simulink model "xianbolvvo2021b"  (R2021b)
settings: Solver=ode1  StartTime=0.0  StopTime=10  FixedStep=0.001  RelTol=1e-3
undefined symbols (not defined in the file): alldata3K_input, alldata3K_output, alldata5K_input, alldata5K_output, alldata7K_input, alldata7K_output, DiscIntNeverNeededParam, Hzden, Hznum
libraries: eeGeneralControl x7, cstblocks x1
settings Model: Creator=renjianze  LastModifiedBy=renjianze
settings DebuggingCC: UnconnectedInputMsg=none  UnconnectedOutputMsg=none  UnconnectedLineMsg=none
settings ModelReferenceCC: EnableRefExpFcnMdlSchedulingChecks=off
settings RTWCC: DLArmComputeVersion=20.02.1

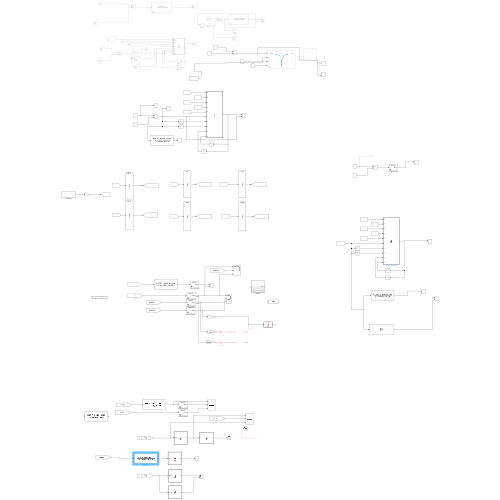
[thumbnail: Simulink's stored preview of the top-level diagram]
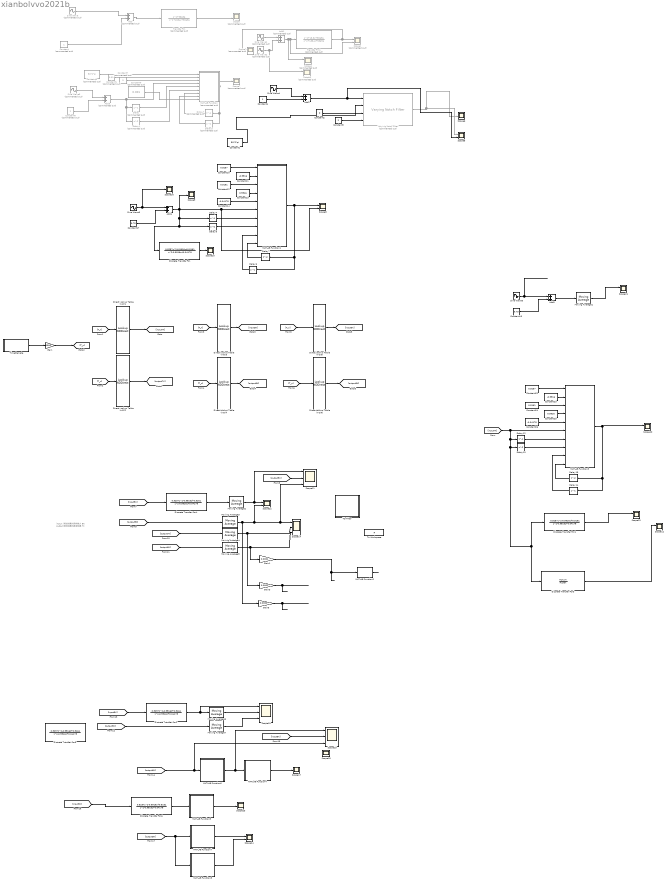
== system xianbolvvo2021b ==
  note: input：测试结果的采样输入 6K
      | output:测试结果的滤波结果  7k
  Add : Sum  Commented=on
  Add1 : Sum  Commented=on
  Add2 : Sum
  Add3 : Sum  Commented=on
  Add4 : Sum
  Add5 : Sum
  Constant : Constant  Commented=on
  Constant1 : Constant  Value=50*2*pi
  Constant10 : Constant  Value=0.5257
  Constant11 : Constant  Value=-0.9916
  Constant12 : Constant  Value=0.5161
  Constant13 : Constant  Value=0.9916
  Constant14 : Constant  Value=-0.04178
  Constant15 : Constant  Value=9.75
  Constant17 : Constant  Value=9.75
  Constant2 : Constant  Value=0
  Constant22 : Constant  Value=0.5257
  Constant23 : Constant  Value=-0.9916
  Constant24 : Constant  Value=0.5161
  Constant25 : Constant  Value=0.9916
  Constant26 : Constant  Value=-0.04178
  Constant3 : Constant  Value=2
  Constant4 : Constant
  Constant5 : Constant  Commented=on  Value=50*2*pi
  Constant6 : Constant  Commented=on  Value=0.01
  Constant7 : Constant  Commented=on  Value=3
  Constant8 : Constant  Commented=on
  Constant9 : Constant  Commented=on  Value=0.001
  Delay : Delay  Commented=on  DelayLength=1
  Delay1 : Delay  Commented=on
  Delay{4,6,12,14} (4 alike) : Delay  DelayLength=1
  Delay{5,7,13,15} (4 alike) : Delay
  Delay2 : Delay  Commented=on  DelayLength=1
  Delay3 : Delay  Commented=on
  Direct Lookup Table (n-D)1 : LookupNDDirect  NumberOfTableDimensions=1  Table=alldata7K_input
  Direct Lookup Table (n-D)2 : LookupNDDirect  NumberOfTableDimensions=1  Table=alldata7K_output
  Direct Lookup Table (n-D)3 : LookupNDDirect  NumberOfTableDimensions=1  Table=alldata5K_input
  Direct Lookup Table (n-D)4 : LookupNDDirect  NumberOfTableDimensions=1  Table=alldata5K_output
  Direct Lookup Table (n-D)5 : LookupNDDirect  NumberOfTableDimensions=1  Table=alldata3K_input
  Direct Lookup Table (n-D)6 : LookupNDDirect  NumberOfTableDimensions=1  Table=alldata3K_output
  Discrete Transfer Fcn{,1..2,4..6} (6 alike) : DiscreteTransferFcn  Numerator=[0.5257 -0.9916 0.5161]  Denominator=[1 -0.9916 0.04178]
  Discrete Transfer Fcn3 : DiscreteTransferFcn  Numerator=Hznum  Denominator=Hzden
  Gain : Gain  Gain=1000
  Gain1 : Gain  Gain=0.0001
  Gain3 : Gain  Gain=0.0001
  Gain5 : Gain  Gain=0.0001
  MATLAB Function : MATLAB Function  Commented=on  TreatAsAtomicUnit=on
  MATLAB Function1 : MATLAB Function  TreatAsAtomicUnit=on
  MATLAB Function2 : MATLAB Function  TreatAsAtomicUnit=on
  MATLAB Function3 : MATLAB Function  TreatAsAtomicUnit=on
  MATLAB Function4 : MATLAB Function  TreatAsAtomicUnit=on
  MATLAB Function5 : MATLAB Function  TreatAsAtomicUnit=on
  MATLAB Function6 : MATLAB Function  TreatAsAtomicUnit=on
  MATLAB Function7 : MATLAB Function  TreatAsAtomicUnit=on
  MATLAB Function8 : MATLAB Function  TreatAsAtomicUnit=on
  Moving Average{1..7} (7 alike) : eeGeneralControl/Moving Average  VariantControl=Variant1  LabelModeActiveChoice=Discrete  f=50  x0=0  BufferSize=8192  Ts=0.001
      settings: SourceProductBaseCode=PS
  Scope{,1..4} (5 alike) : Scope  Commented=on  NumInputPorts=2
  Scope{6,9..10,16..18,23} (7 alike) : Scope
  Scope{11,14..15,19} (4 alike) : Scope  NumInputPorts=3
  Scope{5,8,12..13,20..22,24} (8 alike) : Scope  NumInputPorts=2
  Scope7 : Scope  Commented=on
  Sine Wave : Sin  Commented=on  Amplitude=0.3  Frequency=50*2*pi  SampleTime=0
  Sine Wave1 : Sin  Commented=on  Frequency=50*2*pi  SampleTime=0
  Sine Wave2 : Sin  Commented=on  Frequency=100*2*pi  SampleTime=0
  Sine Wave3 : Sin  Commented=on  Amplitude=0.3  Frequency=50*2*pi  SampleTime=0
  Sine Wave4 : Sin  Amplitude=0.3  Frequency=50*2*pi  SampleTime=0
  Sine Wave5 : Sin  Amplitude=1.25  Frequency=50*2*pi  Phase=pi/2  SampleTime=0
  Sine Wave6 : Sin  Amplitude=1.25  Frequency=50*2*pi  Phase=pi/2  SampleTime=0
  TD Filter : Subsystem
  TimeGenrate : Subsystem
  To Workspace : ToWorkspace  VariableName=R  SampleTime=-1
  Transfer Fcn : TransferFcn  Commented=on  Numerator=[1 0 98696]  Denominator=[1 1884 98696]
  Transfer Fcn1 : TransferFcn  Commented=on  Numerator=[1 18.8 98696]  Denominator=[1 1884 98696]
  Varying Notch Filter : cstblocks/Linear Parameter Varying/Varying Notch Filter  Commented=on
      settings: SourceProductBaseCode=CT
  wires:
  Transfer Fcn/1 -> Scope/2
  Sine Wave/1 -> Add/1
  Constant/1 -> Add/2
  Add/1 -> Transfer Fcn/1
  Sine Wave1/1 -> Add1/1
  Add1/1 -> Scope4/1, Scope1/2, Transfer Fcn1/1
  Transfer Fcn1/1 -> Scope2/1, Scope1/1
  Sine Wave2/1 -> Scope3/1, Add1/2
  Constant1/1 -> Varying Notch Filter/2
  Constant2/1 -> Varying Notch Filter/3
  Constant3/1 -> Varying Notch Filter/4
  Varying Notch Filter/1 -> Scope6/1, Scope5/1
  Sine Wave4/1 -> Add2/1
  Add2/1 -> Scope5/2, Varying Notch Filter/1
  Constant4/1 -> Add2/2
  Constant5/1 -> MATLAB Function/1(freq)
  Constant6/1 -> MATLAB Function/2(gmin)
  Constant7/1 -> MATLAB Function/3(damp)
  Constant8/1 -> Add3/2
  Sine Wave3/1 -> Add3/1
  Add3/1 -> Delay1/1, Delay/1, MATLAB Function/4(x)
  Delay/1 -> MATLAB Function/5(x1)
  Delay1/1 -> MATLAB Function/6(x2)
  MATLAB Function/1(y) -> Delay3/1, Delay2/1, Scope7/1
  Delay2/1 -> MATLAB Function/7(y1)
  Delay3/1 -> MATLAB Function/8(y2)
  Constant9/1 -> MATLAB Function/9(Ts)
  Constant10/1 -> MATLAB Function1/1(a0)
  Constant11/1 -> MATLAB Function1/2(a1)
  Constant12/1 -> MATLAB Function1/3(a2)
  Constant13/1 -> MATLAB Function1/4(b1)
  Constant14/1 -> MATLAB Function1/5(b2)
  Add4/1 -> Scope9/1, Discrete Transfer Fcn/1, Delay5/1, Delay4/1, MATLAB Function1/6(x), Scope8/2
  Sine Wave5/1 -> Scope16/1, Add4/1
  Constant17/1 -> Add4/2
  Delay4/1 -> MATLAB Function1/7(x1)
  Delay5/1 -> MATLAB Function1/8(x2)
  Delay6/1 -> MATLAB Function1/9(y1)
  Delay7/1 -> MATLAB Function1/10(y2)
  MATLAB Function1/1(y) -> Scope8/1, Delay6/1, Delay7/1
  Discrete Transfer Fcn/1 -> Scope10/1
  TimeGenrate/1(t) -> Gain/1
  Gain/1 -> [T_n]
  Direct Lookup Table (n-D)1/1 -> [input7K]
  Direct Lookup Table (n-D)2/1 -> [output7K]
  MATLAB Function3/1(y) -> Scope20/1, Delay15/1, Delay14/1
  Delay15/1 -> MATLAB Function3/10(y2)
  Delay14/1 -> MATLAB Function3/9(y1)
  Delay13/1 -> MATLAB Function3/8(x2)
  Delay12/1 -> MATLAB Function3/7(x1)
  [input7K] -> Delay12/1, Discrete Transfer Fcn1/1, Discrete Transfer Fcn3/1, Delay13/1, MATLAB Function3/6(x)
  Constant26/1 -> MATLAB Function3/5(b2)
  Constant25/1 -> MATLAB Function3/4(b1)
  Constant24/1 -> MATLAB Function3/3(a2)
  Constant23/1 -> MATLAB Function3/2(a1)
  Constant22/1 -> MATLAB Function3/1(a0)
  Discrete Transfer Fcn3/1 -> Scope12/1
  Discrete Transfer Fcn1/1 -> Scope13/1
  Constant15/1 -> Add5/2
  Sine Wave6/1 -> Add5/1
  Add5/1 -> Moving Average1/1
  Moving Average1/1 -> Scope21/1
  Discrete Transfer Fcn4/1 -> Moving Average2/1
  [input5K] -> Discrete Transfer Fcn4/1
  [output5K] -> Moving Average3/1
  Moving Average2/1 -> Scope11/1, Scope22/1
  Moving Average3/1 -> Scope14/1, Scope11/3, Scope22/2, Gain5/1  "nfilter_t"
  [T_n] -> Direct Lookup Table (n-D)1/1
  [T_n] -> Direct Lookup Table (n-D)2/1
  [T_n] -> Direct Lookup Table (n-D)3/1
  [T_n] -> Direct Lookup Table (n-D)4/1
  [T_n] -> Direct Lookup Table (n-D)6/1
  [T_n] -> Direct Lookup Table (n-D)5/1
  Direct Lookup Table (n-D)3/1 -> [input5K]
  Direct Lookup Table (n-D)4/1 -> [output5K]
  Direct Lookup Table (n-D)5/1 -> [input3K]
  Direct Lookup Table (n-D)6/1 -> [output3K]
  [output5K] -> Scope11/2
  [output7K] -> Moving Average4/1
  [output3K] -> Moving Average5/1
  Moving Average4/1 -> Gain3/1, Scope14/2  "nfilter_t"
  Moving Average5/1 -> Gain1/1, Scope14/3  "nfilter_t"
  MATLAB Function2/1(y) -> ?
  Gain1/1 -> MATLAB Function2/1(u)
  Gain3/1 -> ?
  ? -> ?
  Gain5/1 -> ?
  ? -> ?
  [input5K] -> Discrete Transfer Fcn2/1
  Discrete Transfer Fcn2/1 -> Scope19/1, Moving Average6/1
  Moving Average6/1 -> Scope19/2
  [output5K] -> Moving Average7/1
  Moving Average7/1 -> Scope19/3
  [output5K] -> MATLAB Function6/1(FilterIn), Scope15/3
  MATLAB Function6/1(out) -> Scope15/1, MATLAB Function4/1(u)
  MATLAB Function4/1(y) -> Scope17/1
  [input5K] -> Scope15/2
  ? -> Scope18/1
  Discrete Transfer Fcn6/1 -> MATLAB Function5/1(FilterIn)
  [input5K] -> Discrete Transfer Fcn6/1
  MATLAB Function5/1(out) -> Scope23/1
  [output5K] -> MATLAB Function8/1(FilterIn), MATLAB Function7/1(FilterIn)
  MATLAB Function7/1(out) -> Scope24/1
  MATLAB Function8/1(out) -> Scope24/2

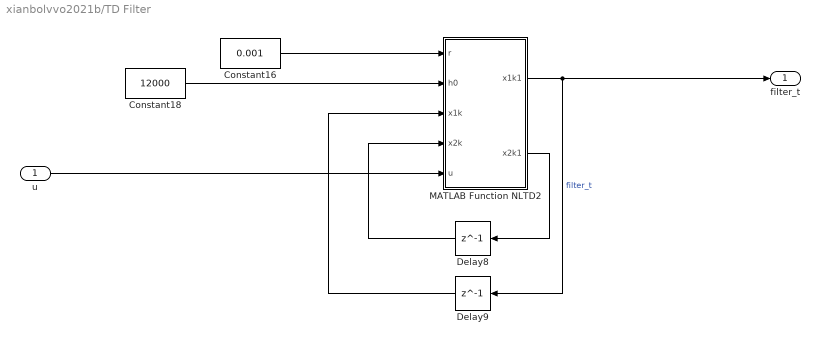
== system xianbolvvo2021b/TD Filter ==
  u : Inport
  Constant16 : Constant  Value=0.001
  Constant18 : Constant  Value=12000
  Delay8 : Delay  DelayLength=1
  Delay9 : Delay  DelayLength=1
  MATLAB Function NLTD2 : MATLAB Function  TreatAsAtomicUnit=on
  filter_t : Outport
  wires:
  Delay9/1 -> MATLAB Function NLTD2/3(x1k)
  u/1 -> MATLAB Function NLTD2/5(u)
  Constant16/1 -> MATLAB Function NLTD2/1(r)
  MATLAB Function NLTD2/1(x1k1) -> filter_t/1, Delay9/1  "filter_t"
  Constant18/1 -> MATLAB Function NLTD2/2(h0)
  Delay8/1 -> MATLAB Function NLTD2/4(x2k)
  MATLAB Function NLTD2/2(x2k1) -> Delay8/1

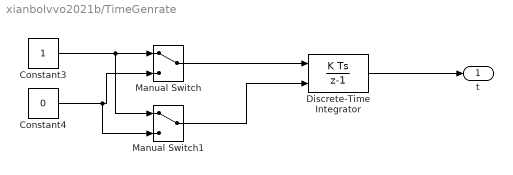
== system xianbolvvo2021b/TimeGenrate ==
  Constant3 : Constant
  Constant4 : Constant  Value=0
  Discrete-Time Integrator : DiscreteIntegrator  ExternalReset=either  SampleTime=-1  ICPrevOutput=DiscIntNeverNeededParam  ICPrevScaledInput=DiscIntNeverNeededParam
  Manual Switch : ManualSwitch
  Manual Switch1 : ManualSwitch
  t : Outport
  wires:
  Constant3/1 -> Manual Switch1/1, Manual Switch/1
  Constant4/1 -> Manual Switch1/2, Manual Switch/2
  Manual Switch1/1 -> Discrete-Time Integrator/2
  Discrete-Time Integrator/1 -> t/1
  Manual Switch/1 -> Discrete-Time Integrator/1

== matlab function xianbolvvo2021b/TD Filter/MATLAB Function NLTD2 ==
  data: r input; h0 input; x1k input; x2k input; u input; x1k1 output size=1; x2k1 output size=1
function [x1k1,x2k1] = fcn(r,h0,x1k,x2k,u)

fh = fst(x1k, x2k,u, r, h0);

x1k1 = x1k+h0*x2k;
x2k1 = x2k+h0*fh;

== matlab function xianbolvvo2021b/MATLAB Function1 ==
  data: a0 input; y output; a1 input; a2 input; b1 input; b2 input; x input; x1 input; x2 input; y1 input; y2 input
function y = fcn(a0,a1,a2,b1,b2,x,x1,x2,y1,y2)
    


y = a0*x+a1*x1+a2*x2+b1*y1+b2*y2;

== matlab function xianbolvvo2021b/MATLAB Function ==
  data: freq input; y output; gmin input; damp input; x input; x1 input; x2 input; y1 input; y2 input; Ts input
function y = fcn(freq,gmin,damp,x,x1,x2,y1,y2,Ts)
    
    a1 = 2 + 2*damp*freq*Ts;
    a2 = 1 -2 *damp * freq *Ts + freq*freq*Ts*Ts;
    b0 = 1;
    b1 = 2+2*gmin*damp*freq*Ts;
    b2 = 1-2*gmin*damp*freq *Ts + freq*freq*Ts*Ts;

y = b0*x+b1*x1+b2*x2-a1*y1-a2*y2;

== matlab function xianbolvvo2021b/MATLAB Function2 ==
  data: u input; y output
function y = fcn(u)
u = 0.0001*u;
y = -(3569184000000000000*u-5885584000000000000)/(338160000000*u-933625800000);
y = y*0.001;

== matlab function xianbolvvo2021b/MATLAB Function3 ==
  data: a0 input; y output; a1 input; a2 input; b1 input; b2 input; x input; x1 input; x2 input; y1 input; y2 input
function y = fcn(a0,a1,a2,b1,b2,x,x1,x2,y1,y2)
    


y = a0*x+a1*x1+a2*x2+b1*y1+b2*y2;

== matlab function xianbolvvo2021b/MATLAB Function4 ==
  data: u input; y output
function y = fcn(u)
u = 0.0001*u;
y = -(3569184000000000000*u-5885584000000000000)/(338160000000*u-933625800000);
y = y*0.001;

== matlab function xianbolvvo2021b/MATLAB Function5 ==
  data: FilterIn input; out output
function out = fcn(FilterIn)
% 需要修改采样时间和过滤的频率
% sample = 0.001;
% fre = 50;
% n = uint16( 1/(sample*fre));

persistent Temp;

if isempty(Temp)
    Temp = zeros(20,1);
end

Temp = [Temp(2:20); FilterIn];
out = ( sum(Temp) - min(Temp) -max(Temp)  )/18;
% out =mean(Temp);

end

== matlab function xianbolvvo2021b/MATLAB Function6 ==
  data: FilterIn input; out output
function out = fcn(FilterIn)
% 需要修改采样时间和过滤的频率
sample = 0.001;
fre = 50;
n = uint16( 1/(sample*fre));

persistent Temp;

if isempty(Temp)
    Temp = zeros(n,1);
end

Temp = [Temp(2:20); FilterIn];
out =mean(Temp);

end

== matlab function xianbolvvo2021b/MATLAB Function7 ==
  data: FilterIn input; out output
function out = fcn(FilterIn)
% 需要修改采样时间和过滤的频率
% sample = 0.001;
% fre = 50;
% n = uint16( 1/(sample*fre));

persistent Temp;

if isempty(Temp)
    Temp = zeros(20,1);
end

Temp = [Temp(2:20); FilterIn];
out = ( sum(Temp) - min(Temp) -max(Temp)  )/18;
% out =mean(Temp);

end

== matlab function xianbolvvo2021b/MATLAB Function8 ==
  data: FilterIn input; out output
function out = fcn(FilterIn)
% 需要修改采样时间和过滤的频率
sample = 0.001;
fre = 50;
n = uint16( 1/(sample*fre));

persistent Temp;

if isempty(Temp)
    Temp = zeros(n,1);
end

Temp = [Temp(2:20); FilterIn];
out =mean(Temp);

end
